simulink model "part2"  (R2020a)
settings: Solver=FixedStepAuto  StartTime=0.0  StopTime=150  FixedStep=0.1  RelTol=1e-3
values from neighbouring files (symbols this model uses):
  A = [zeros(3), eye(3) ... (first row only)    [initEKF.m]    (also in initEKF.mat = [0 0 0 -0.394784176044 0 0 0 0 0 0 -0.394784176044 0 ... (36)
  B = [0 0 0 0 0 0 1.46677031844e-07 0 0 0 0 0 ... (27 elements, 9x3)]    [ExtendedKalmanFilter.mat]    (also in initEKF.m = [zeros(6,3); initEKF.mat = [0 0 0 0 0 0 0 0 0 0 0 0 ... (45 elements, 15x3)]; initObserverInput.m = [zeros(6,3);zeros(3,3);zeros(3,3);invM]; initObserverInput.mat = [0 0 0 0 0 0 0 0 0 0 0 0 ... (45 elements, 15x3)])
  ConstSPSuge = 0    [ExtendedKalmanFilter.mat]    (also in doSimPart2.m; init.m; init1.m; init_weather.m)
  ConstSPSway = 0    [ExtendedKalmanFilter.mat]    (also in doSimPart2.m; init.m; init1.m; init_weather.m)
  ConstSPYaw = 0    [ExtendedKalmanFilter.mat]    (also in doSimPart2.m; init.m; init1.m; init_weather.m)
  Curent_Slaw_var = 0    [ExtendedKalmanFilter.mat]    (also in doSimPart2.m; init.m; init1.m; init_weather.m = 1)
  Current_Head_mu = 0.001    [ExtendedKalmanFilter.mat]    (also in doSimPart2.m; init.m; init1.m; init_weather.m)
  Current_Head_Sample_time = 1    [ExtendedKalmanFilter.mat]    (also in doSimPart2.m; init.m; init1.m; init_weather.m)
  Current_input_type = 0    [ExtendedKalmanFilter.mat]    (also in doSimPart2.m; init.m; init1.m; init_weather.m)
  Current_Speed = 0    [ExtendedKalmanFilter.mat]    (also in doSimPart2.m = 0.2; init.m; init1.m; init_weather.m = 0.2)
  CurrHead =     [ExtendedKalmanFilter.mat]
  D = [264860  0  0; 0  881640  0; 0  0  337740000]    [ExtendedKalmanFilter.mat]    (also in initEKF.m = [2.6486e5, 0, 0; initEKF.mat; initObserverInput.m = diag([2.6486e5, 8.8164e5, 3.3774e8]); initObserverInput.mat)
  E = [0 0 0 1 0 0 0 0 0 0 0 0 ... (27 elements, 9x3)]    [ExtendedKalmanFilter.mat]    (also in initEKF.m = [Ew, zeros(6,3); initEKF.mat = [0 0 0 0.01 0 0 0 0 0 0 0 0 ... (90 elements, 15x6)]; initObserverInput.m = [Ew, zeros(6,3); zeros(3), zeros(3); zeros(3), Eb; zeros(3),; initObserverInput.mat = [0 0 0 0.01 0 0 0 0 0 0 0 0 ... (90 elements, 15x6)])
  H = [1 0 0 0 1 0 0 0 1 0 0 0 ... (27 elements, 3x9)]    [ExtendedKalmanFilter.mat]    (also in initEKF.m = [C, eye(3), zeros(3), zeros(3)]; initEKF.mat = [0 0 0 0 0 0 0 0 0 1 0 0 ... (45 elements, 3x15)]; initObserverInput.m = [Cw, eye(3), zeros(3), zeros(3)]; initObserverInput.mat = [0 0 0 0 0 0 0 0 0 1 0 0 ... (45 elements, 3x15)])
  h = polar(Wind_Headind_EF.Data(:,1),Wind_Speed.Data(:,1))    [init.m]    (also in init1.m; initEKF.m = 0.1; initEKF.mat = 0.1; initObserverInput.m = 0.1)
  invM = inv(M)    [initEKF.m]    (also in initEKF.mat = [1.46677031844e-07  0  0; 0  1.2695973473e-07  9.23036390732; initObserverInput.m; initObserverInput.mat = [1.46677031844e-07  0  0; 0  1.2695973473e-07  9.23036390732)
  invT = inv(T)    [initEKF.m]    (also in initEKF.mat = [0.001  0  0; 0  0.001  0; 0  0  0.001])
  Kd_surge = 1868784.40925    [ExtendedKalmanFilter.mat]    (also in doSimPart2.m = 2*0.7*sqrt(6.4794^5+6.362*10^6)*sqrt(Kp_surge); init.m = 2*0.7*sqrt(6.4794^5+6.362*10^6)*sqrt(Kp_surge); init1.m = 2*0.7*sqrt(6.4794^5+6.362*10^6)*sqrt(Kp_surge); init_weather.m = 2*0.7*sqrt(6.4794^5+6.362*10^6)*sqrt(Kp_surge))
  Kd_sway = 3746851.89423    [ExtendedKalmanFilter.mat]    (also in doSimPart2.m = 2*0.7*sqrt(2.157*10^6+6.362*10^6)*sqrt(Kp_sway); init.m = 2*0.7*sqrt(2.157*10^6+6.362*10^6)*sqrt(Kp_sway); init1.m = 2*0.7*sqrt(2.157*10^6+6.362*10^6)*sqrt(Kp_sway); init_weather.m = 2*0.7*sqrt(2.157*10^6+6.362*10^6)*sqrt(Kp_sway))
  Kd_yaw = 3338344318.3    [ExtendedKalmanFilter.mat]    (also in doSimPart2.m = 2*0.7*sqrt(1.0711*10^9+2.724*10^9)*sqrt(Kp_yaw); init.m = 2*0.7*sqrt(1.0711*10^9+2.724*10^9)*sqrt(Kp_yaw); init1.m = 2*0.7*sqrt(1.0711*10^9+2.724*10^9)*sqrt(Kp_yaw); init_weather.m = 2*0.7*sqrt(1.0711*10^9+2.724*10^9)*sqrt(Kp_yaw))
  Ki_surge = 18000    [ExtendedKalmanFilter.mat]    (also in doSimPart2.m; init.m; init1.m; init_weather.m)
  Ki_sway = 80000    [ExtendedKalmanFilter.mat]    (also in doSimPart2.m; init.m; init1.m; init_weather.m)
  Ki_yaw = 150000000    [ExtendedKalmanFilter.mat]    (also in doSimPart2.m; init.m; init1.m; init_weather.m = 150000)
  Kp_surge = 279569.493868    [ExtendedKalmanFilter.mat]    (also in doSimPart2.m; init.m; init1.m; init_weather.m = 195698.645708)
  Kp_sway = 840791.598929    [ExtendedKalmanFilter.mat]    (also in doSimPart2.m; init.m; init1.m; init_weather.m = 588554.11925)
  Kp_yaw = 1498245426.5    [ExtendedKalmanFilter.mat]    (also in doSimPart2.m; init.m; init1.m; init_weather.m = 104877179.855)
  p_bar = zeros(15)    [initEKF.m]    (also in initEKF.mat = [0 0 0 0 0 0 0 0 0 0 0 0 ... (225 elements, 15x15)])
  Q = [1000000000000  0  0; 0  1000000000000  0; 0  0  100000000000000]    [ExtendedKalmanFilter.mat]    (also in initEKF.m = [10^4, 0, 0, 0, 0, 0; initEKF.mat = [10000 0 0 0 0 0 0 10000 0 0 0 0 ... (36 elements, 6x6)]; initObserverInput.m = diag([ 10^4 10^4 10^3 10^9 10^9 10^9]); initObserverInput.mat = [10000 0 0 0 0 0 0 10000 0 0 0 0 ... (36 elements, 6x6)])
  R = [1.15e-05  0  0; 0  1.2e-06  0; 0  0  4e-08]    [ExtendedKalmanFilter.mat]    (also in initEKF.m = [1, 0,0; initEKF.mat = [1  0  0; 0  1  0; 0  0  0.1]; initObserverInput.m = diag([1,1,0.1]); initObserverInput.mat = [1  0  0; 0  1  0; 0  0  0.1])
  thrusters =     [ExtendedKalmanFilter.mat]
  typeOfSimulation = 2    [ExtendedKalmanFilter.mat]    (also in doSimPart2.m = 0; init.m; init1.m; init_weather.m)
  vessel =     [ExtendedKalmanFilter.mat]
  Wind_gust_k = 0.0026    [ExtendedKalmanFilter.mat]    (also in doSimPart2.m; init.m; init1.m; init_weather.m)
  Wind_gust_L = 1800    [ExtendedKalmanFilter.mat]    (also in doSimPart2.m; init.m; init1.m; init_weather.m)
  Wind_gust_nfreq = 1000    [ExtendedKalmanFilter.mat]    (also in doSimPart2.m; init.m; init1.m; init_weather.m)
  Wind_gust_phi = [1.94720348827 2.24175439974 2.07841268688 2.94269508899 2.5189968857 3.92559282604 1.02965824361 5.79326836705 3.39416152385 6.24100933894 1.9296881265 4.15801677987 ... (1000 elements, 1000x1)]    [ExtendedKalmanFilter.mat]    (also in doSimPart2.m = 2*pi * rand(Wind_gust_nfreq,1); init.m = 2*pi * rand(Wind_gust_nfreq,1); init1.m = 2*pi * rand(Wind_gust_nfreq,1); init_weather.m = 2*pi * rand(Wind_gust_nfreq,1))
  Wind_Gust_type = 0    [ExtendedKalmanFilter.mat]    (also in doSimPart2.m = 1; init.m; init1.m; init_weather.m = 1)
  Wind_Head_mean = 1.57079632679    [ExtendedKalmanFilter.mat]    (also in doSimPart2.m = vector_Headings_rad; init.m; init1.m; init_weather.m = 0)
  Wind_Head_mu = 0.001    [ExtendedKalmanFilter.mat]    (also in doSimPart2.m; init.m; init1.m; init_weather.m)
  Wind_Head_Sample_time = 1    [ExtendedKalmanFilter.mat]    (also in doSimPart2.m; init.m; init1.m; init_weather.m)
  Wind_Heading_type = 0    [ExtendedKalmanFilter.mat]    (also in doSimPart2.m; init.m; init1.m; init_weather.m = 1)
  Wind_U10 = 0    [ExtendedKalmanFilter.mat]    (also in doSimPart2.m = 15; init.m; init1.m; init_weather.m)
  Wind_U_mean = 0    [ExtendedKalmanFilter.mat]    (also in doSimPart2.m = Umean; init.m = Umean; init1.m = Umean; init_weather.m = Umean)
  Wind_U_mu = 0.001    [ExtendedKalmanFilter.mat]    (also in doSimPart2.m; init.m; init1.m; init_weather.m)
  Wind_U_Sample_time = 1    [ExtendedKalmanFilter.mat]    (also in doSimPart2.m; init.m; init1.m; init_weather.m)
  Wind_U_type = 0    [ExtendedKalmanFilter.mat]    (also in doSimPart2.m = 1; init.m; init1.m; init_weather.m = 1)
  x_bar = zeros(15,1)    [initEKF.m]    (also in initEKF.mat = [0 0 0 0 0 0 0 0 0 0 0 0 ... (15 elements, 15x1)])
undefined symbols (not defined in the file or in its folder): Hoerner
libraries: marine_gnc x10, simulink x4, marine_hydro x2
(part 2 of 2)

== matlab function part2/Thrust Allocation/MATLAB Function ==
  data: u_l input; u output; tau_c input; alpha output; alpha_l input; clock input; clock_l input
function [u, alpha] = Thruster_allocation(u_l, tau_c, alpha_l, clock, clock_l)

x1=39.3; x2=35.3; x3=31.3; x4=-28.5; x5=x4; %assigning x values
y4=5; y5=-5; %assigning y values

B_9=[0   1   0   1   0   1   0   1   0;...
     1   0   1   0   1   0   1   0   1;...
    x1  0   x2  0   x3 -y4  x4 -y5  x5];

[m, p]=size(B_9); %m is DOF, p is number of thursters
f_r=2; %define the radius of forbidden sector from forbidden radius of the influenced propeller
w=eye(m);

dt=clock-clock_l;
%dt=1;

u_cons=[125000; 150000; 150000; 320000; 320000];
u1=zeros(p,1); alpha=zeros(5,1); alpha(1)=pi/2; incl=ones(5,1);
u_C=zeros(9,1); u_Ci=zeros(5,1); usat=zeros(5,1); B9_c=zeros(m,p);
usatu=zeros(9,1); utot=zeros(5,1); tau_test=zeros(3,1); u=zeros(5,1);
B9_u=zeros(m,p); u_negative_check=zeros(5, 1); u_n=zeros(9,1);
noofrate9=zeros(9,1);

%rate changes
a_rate=4*pi/60*dt; %alpha, same for all azimuths
T_rate=[1/8 1/8 1/8 1/10 1/10]*dt; %rate change thrusters, must be multiplied by max torque

%forbidden sectors, [lower bounds, upperbounds], alpha=[alpha_2 alpha_3 alpha_4 alpha_5] 
a_1_for=[0 0];
a_2_for=[pi-atan(f_r/4) pi+atan(f_r/4)]; 
a_3_for=[atan(f_r/4) 2*pi-atan(f_r/4)]; 
a_4_for=[3*pi/2-atan(f_r/10) 3*pi/2+atan(f_r/10)];
a_5_for=[pi/2-atan(f_r/10) pi/2+tan(f_r/10)];
alph=[a_1_for; a_2_for; a_3_for; a_4_for; a_5_for];

% wl=1;
% e=10^-3;

C=pinv(B_9);
u1=C*tau_c;
itr=1;

counter=0;


while itr==1
    itr=0;

    counter=counter+1;    
    
    %calculate new alpha
    k=1;
    %from u in 9x1 to alpha and u 5x1
    utot(1)=u1(1);
    [alpha(2), utot(2)]=cart2pol(u1(2,1), u1(3,1));
    [alpha(3), utot(3)]=cart2pol(u1(4,1), u1(5,1));
    [alpha(4), utot(4)]=cart2pol(u1(6,1), u1(7,1));
    [alpha(5), utot(5)]=cart2pol(u1(8,1), u1(9,1));
    
    %checking alpha rate constraint
    new=0;
    for i=2:length(alpha) 
            if alpha(i)-alpha_l(i)>a_rate
                alpha(i)=alpha_l(i)+a_rate;
                new=1;
            elseif alpha_l(i)-alpha(i)>a_rate
                alpha(i)=alpha_l(i)-a_rate;
                new=1;
            end
    end
    if new==1
        B=[0 cos(alpha(2)) cos(alpha(3)) cos(alpha(4)) cos(alpha(5));...
           1 sin(alpha(2)) sin(alpha(3)) sin(alpha(4)) sin(alpha(5));...
           x1 x2*sin(alpha(2)) x3*sin(alpha(3)) x4*sin(alpha(4))-y4*cos(alpha(4)) x5*sin(alpha(5))-y5*cos(alpha(5))];
        C5=pinv(B);
        u5=C5*tau_c;
%         for j=1:length(u5)
%             if u5(j)<0
%                 u5(j)=0;
%                 utot(j)=0;
%             end
%         end
        utot=u5;
    end
        
    %calculate if above truster rate and correct if so
    noofrate=zeros(5,1);    
    for i=1:length(utot)
        if utot(i)-u_l(i)>T_rate(i)*u_cons(i)
            utot(i)=u_l(i)+T_rate(i)*u_cons(i);
            u_Ci(i)=u_l(i)+T_rate(i)*u_cons(i);
            noofrate(i)=1; %1 indicate that it cannot be increased
        elseif u_l(i)-utot(i)>T_rate(i)*u_cons(i)
            utot(i)=u_l(i)-T_rate(i)*u_cons(i);
            u_Ci(i)=u_l(i)-T_rate(i)*u_cons(i);
            noofrate(i)=1; %1 indicate that it cannot be increased
        end
    end
    if utot(1)-u_l(1)>T_rate(1)
        utot(1)=u_l(1)+T_rate(1)*u_cons(1);
        u_Ci(1)=utot(1);
        noofrate(1)=1;
    elseif u_l(1)-utot(1)>T_rate(1)
        utot(1)=u_l(1)-T_rate(1)*u_cons(1);
        u_Ci(1)=utot(1);
        noofrate(1)=1;
    end     
    
    if sum(noofrate)==5 %if all thruster rates are exceeded
        u=utot;
        itr=0;
    end
    
    %check if saturated thruster
    usat=zeros(5,1);
    if abs(utot(1))>u_cons(1)
        utot(1)=sign(utot(1))*u_cons(1);
        u_Ci(1)=utot(1);
        usat(1)=1;
    end
    for i=2:length(utot)
        if utot(i)>u_cons(i) %if thruster is more than allowed, thrust is set to max
            utot(i)=u_cons(i);
            usat(i)=1;
            u_Ci(i)=u_cons(i);
        else
            u_Ci(i)=utot(i);
        end
    end
    %check max
    u_C(1)=u_Ci(1); 
    u_C(2)=u_Ci(2)*cos(alpha(2)); u_C(3)=u_Ci(2)*sin(alpha(2)); usatu(2)=usat(2); usatu(3)=usat(2);
    u_C(4)=u_Ci(3)*cos(alpha(3)); u_C(5)=u_Ci(3)*sin(alpha(3)); usatu(4)=usat(3); usatu(5)=usat(3);
    u_C(6)=u_Ci(4)*cos(alpha(4)); u_C(7)=u_Ci(4)*sin(alpha(4)); usatu(6)=usat(4); usatu(7)=usat(4);
    u_C(8)=u_Ci(5)*cos(alpha(5)); u_C(9)=u_Ci(5)*sin(alpha(5)); usatu(8)=usat(5); usatu(9)=usat(5);
    noofrate9=[noofrate(1) noofrate(2) noofrate(2) noofrate(3) noofrate(3) noofrate(4) noofrate(4) noofrate(5) noofrate(5)]; 

    for j=1:p
        if usatu(j)==1 || noofrate9(i)==1
            B9_u(1,j)=0; B9_u(2,j)=0; B9_u(3,j)=0;
            B9_c(1,j)=B_9(1,j); B9_c(2,j)=B_9(2,j); B9_c(3,j)=B_9(3,j);
        else
            B9_u(1,j)=B_9(1,j); B9_u(2,j)=B_9(2,j); B9_u(3,j)=B_9(3,j);
            B9_c(1,j)=0; B9_c(2,j)=0; B9_c(3,j)=0;
        end
    end
    allthrustersset=min(noofrate+usat); %adding together so that if all thrusters are maxed out, none will be zero
    if sum(usat)==5
        utot=u_cons;
        itr=0;
    elseif min(allthrustersset)>0
        itr=0;
    elseif sum(usat)>0 && sum(noofrate)>0
        tau_C=B9_c*u_C;
        tau_c=tau_c-tau_C;
        C_new=pinv(B9_u);
        u_n=C_new*tau_c;
        u1=u_C+u_n;
        utot=[u_C(1) sqrt(u_C(2)^2+u_C(3)^2) sqrt(u_C(4)^2+u_C(5)^2) sqrt(u_C(6)^2+u_C(7)^2) sqrt(u_C(8)^2+u_C(9)^2)]';
        itr=1;
    end
    
    if sum(u_n)<100 || sum(u_C)==0
        itr=0;
    end
    

%     if alpha(2)>a_2_for(1) && alpha(2)<a_2_for(2)
%         utot(2)=0;
%     elseif alpha(3)<a_3_for(1) && alpha(3)>a_3_for(2)
%         utot(3)=0;
%     elseif alpha(4)>a_4_for(1) && alpha(4)<a_4_for(2)
%         utot(4)=0;
%     elseif alpha(5)>a_5_for(1) && alpha(5)<a_5_for(2)
%         utot(5)=0;
%     end

    if counter==100
        itr=0;
    end
    
end
    


u=utot;

== matlab function part2/Thruster Dynamics/MATLAB Function ==
  data: alpha_actual input; thrust_actual input; actual_tau output; PosX input; PosY input
function actual_tau   = fcn(alpha_actual,thrust_actual,PosX,PosY)

    Alpha_surge =[cos(alpha_actual(1)) cos(alpha_actual(2)) cos(alpha_actual(3)) cos(alpha_actual(4)) cos(alpha_actual(5))];  
    Alpha_sway = [sin(alpha_actual(1)) sin(alpha_actual(2)) sin(alpha_actual(3)) sin(alpha_actual(4)) sin(alpha_actual(5))];
    Alpha_yaw = [sin(alpha_actual(1))*PosX(1)-cos(alpha_actual(1))*PosY(1) sin(alpha_actual(2))*PosX(2)-cos(alpha_actual(2))*PosY(2) ...
                 sin(alpha_actual(3))*PosX(3)-cos(alpha_actual(3))*PosY(3) sin(alpha_actual(4))*PosX(4)-cos(alpha_actual(4))*PosY(4) ...
                 sin(alpha_actual(5))*PosX(5)-cos(alpha_actual(5))*PosY(5)];

    actual_tau = [Alpha_surge; Alpha_sway; Alpha_yaw]*thrust_actual;
end
